simulink model "beta_inte"  (R2016b)
settings: Solver=FixedStepAuto  StartTime=0.0  StopTime=90  FixedStep=0.01  RelTol=1e-3
values from neighbouring files (symbols this model uses):
  T = 0.47    [Init_for_washout_filter.m]
settings Model: Creator=pallavr  LastModifiedBy=pallavr

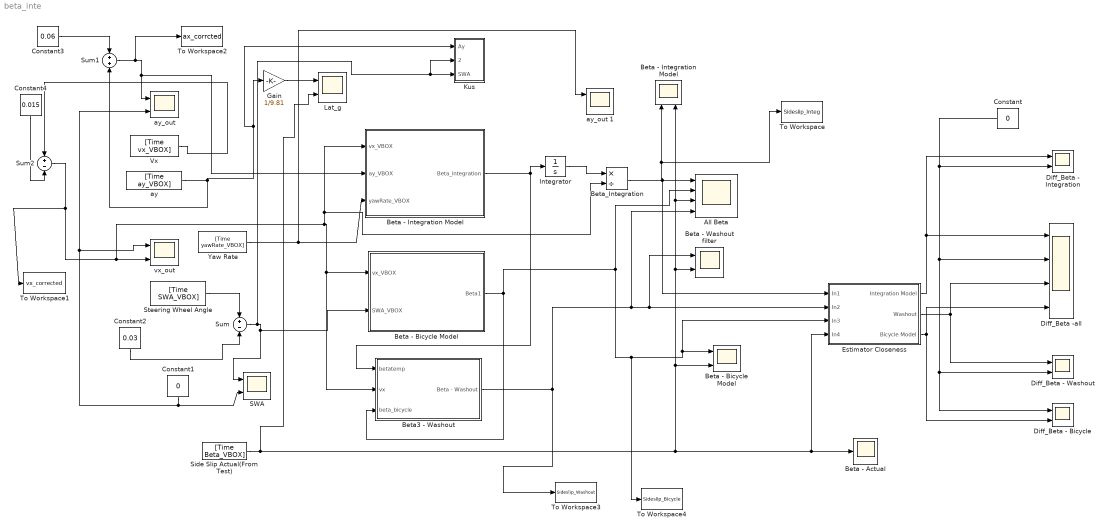
== system beta_inte ==
  " Beta - Bicycle Model" : Scope  NumInputPorts=2
  " Beta - Integration Model" : Scope  NumInputPorts=2
  " Beta - Washout filter" : Scope  NumInputPorts=2
  All Beta : Scope  NumInputPorts=4
  Beta - Actual : Scope
  Beta - Bicycle Model : MATLAB Function  TreatAsAtomicUnit=on
  Beta - Integration Model : MATLAB Function  TreatAsAtomicUnit=on
  "Beta3 - Washout " : Subsystem
  Beta_Integration : Product  Inputs=*/
  Constant : Constant  Value=0
  Constant1 : Constant  Value=0
  Constant2 : Constant  Value=0.03
  Constant3 : Constant  Value=0.06
  Constant4 : Constant  Value=0.015
  "Diff_Beta - Bicycle " : Scope  NumInputPorts=2
  Diff_Beta - Integration : Scope  NumInputPorts=2
  Diff_Beta - Washout : Scope  NumInputPorts=2
  Diff_Beta -all : Scope  NumInputPorts=4
  Estimator Closeness : Subsystem
  Gain : Gain  Gain=1/9.81
  Integrator : Integrator
  Kus : Subsystem
  Lat_g : Scope  NumInputPorts=2
  "SWA " : Scope  NumInputPorts=2
  Side Slip Actual(From Test) : FromWorkspace  VariableName=[Time Beta_VBOX]  SampleTime=0
  Steering Wheel Angle : FromWorkspace  VariableName=[Time SWA_VBOX]  SampleTime=0
  Sum : Sum  Inputs=+-
  Sum1 : Sum
  Sum2 : Sum  Inputs=+-
  To Workspace : ToWorkspace  VariableName=Sideslip_Integ  SampleTime=-1
  To Workspace1 : ToWorkspace  VariableName=vx_corrected  SampleTime=-1
  To Workspace2 : ToWorkspace  VariableName=ax_corrcted  SampleTime=-1
  To Workspace3 : ToWorkspace  VariableName=Sideslip_Washout  SampleTime=-1
  To Workspace4 : ToWorkspace  VariableName=Sideslip_Bicycle  SampleTime=-1
  Vx : FromWorkspace  VariableName=[Time vx_VBOX]  SampleTime=0
  Yaw Rate : FromWorkspace  VariableName=[Time yawRate_VBOX]  SampleTime=0
  ay : FromWorkspace  VariableName=[Time ay_VBOX]  SampleTime=0
  "ay_out " : Scope  NumInputPorts=2
  ay_out 1 : Scope  NumInputPorts=2
  "vx_out " : Scope  NumInputPorts=2
  wires:
  Integrator/1 -> Beta_Integration/1
  Beta - Bicycle Model/1(Beta1) -> Estimator Closeness/3(In3), " Beta - Bicycle Model"/1, To Workspace4/1, All Beta/2, "Beta3 - Washout "/3(beta_bicycle)
  Beta_Integration/1 -> Estimator Closeness/1(In1), All Beta/1, To Workspace/1, " Beta - Integration Model"/1
  Side Slip Actual(From Test)/1 -> Lat_g/2, " Beta - Integration Model"/2, All Beta/3, " Beta - Washout filter"/2, " Beta - Bicycle Model"/2, Beta - Actual/1, Estimator Closeness/4(In4)
  ay/1 -> Kus/1(Ay), Gain/1, Sum1/2
  Yaw Rate/1 -> Beta - Integration Model/3(yawRate_VBOX), ay_out 1/1
  Beta - Integration Model/1(Beta_integration) -> Integrator/1, "Beta3 - Washout "/1(betatemp)
  "Beta3 - Washout "/1(Beta - Washout) -> " Beta - Washout filter"/1, Estimator Closeness/2(In2), All Beta/4, To Workspace3/1
  Estimator Closeness/1(Integration Model) -> Diff_Beta - Integration/1, Diff_Beta -all/1
  Estimator Closeness/2("Washout ") -> Diff_Beta - Washout/1, Diff_Beta -all/3
  Constant/1 -> Diff_Beta - Integration/2, Diff_Beta -all/2, Diff_Beta - Washout/2, "Diff_Beta - Bicycle "/1
  Estimator Closeness/3(Bicycle Model) -> Diff_Beta -all/4, "Diff_Beta - Bicycle "/2
  Gain/1 -> Lat_g/1
  Steering Wheel Angle/1 -> Sum/1
  Constant1/1 -> "SWA "/2, "vx_out "/1, "ay_out "/2
  Vx/1 -> Sum2/1
  Constant2/1 -> Sum/2
  Constant3/1 -> Sum1/1
  Sum1/1 -> To Workspace2/1, Beta - Integration Model/2(ay_VBOX), "ay_out "/1
  Constant4/1 -> Sum2/2
  Sum2/1 -> To Workspace1/1, Beta_Integration/2, Beta - Integration Model/1(vx_VBOX), Beta - Bicycle Model/1(vx_VBOX), "Beta3 - Washout "/2(vx), "vx_out "/2
  Sum/1 -> Kus/2("SWA_in "), Kus/3(SWA), Beta - Bicycle Model/2(SWA_VBOX), "SWA "/1

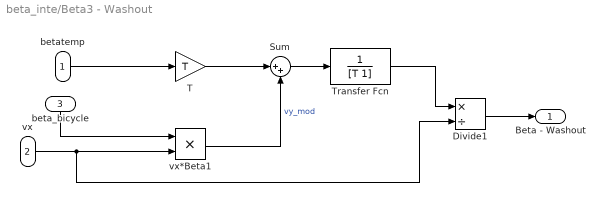
== system beta_inte/Beta3 - Washout  ==
  betatemp : Inport
  vx : Inport  Port=2
  beta_bicycle : Inport  Port=3
  Divide1 : Product  Inputs=*/
  Sum : Sum  Inputs=|++
  T : Gain  Gain=T
  Transfer Fcn : TransferFcn  Denominator=[T 1]
  vx*Beta1 : Product
  Beta - Washout : Outport
  wires:
  Sum/1 -> Transfer Fcn/1
  T/1 -> Sum/1
  Transfer Fcn/1 -> Divide1/1
  Divide1/1 -> Beta - Washout/1
  vx*Beta1/1 -> Sum/2  "vy_mod"
  vx/1 -> Divide1/2, vx*Beta1/2
  beta_bicycle/1 -> vx*Beta1/1
  betatemp/1 -> T/1

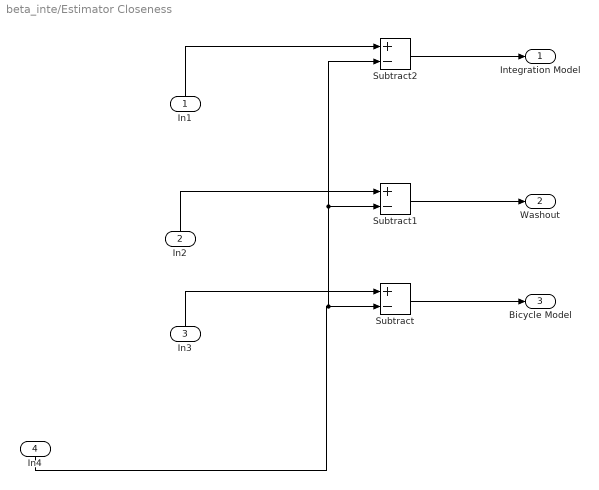
== system beta_inte/Estimator Closeness ==
  In1 : Inport
  In2 : Inport  Port=2
  In3 : Inport  Port=3
  In4 : Inport  Port=4
  Subtract : Sum  Inputs=+-
  Subtract1 : Sum  Inputs=+-
  Subtract2 : Sum  Inputs=+-
  Integration Model : Outport
  "Washout " : Outport  Port=2
  Bicycle Model : Outport  Port=3
  wires:
  Subtract2/1 -> Integration Model/1
  Subtract/1 -> Bicycle Model/1
  In3/1 -> Subtract/1
  In4/1 -> Subtract2/2, Subtract1/2, Subtract/2
  In2/1 -> Subtract1/1
  In1/1 -> Subtract2/1
  Subtract1/1 -> "Washout "/1

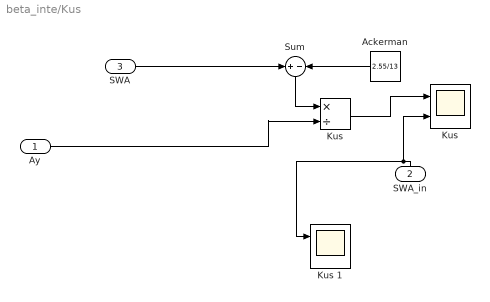
== system beta_inte/Kus ==
  Ay : Inport
  "SWA_in " : Inport  Port=2
  SWA : Inport  Port=3
  Ackerman : Constant  Value=2.55/13
  Kus : Product  Inputs=*/
  "Kus " : Scope  NumInputPorts=2
  Kus 1 : Scope  NumInputPorts=2
  Sum : Sum  Inputs=+-
  wires:
  Ackerman/1 -> Sum/2
  Kus/1 -> "Kus "/1
  Sum/1 -> Kus/1
  SWA/1 -> Sum/1
  Ay/1 -> Kus/2
  "SWA_in "/1 -> "Kus "/2, Kus 1/1

== matlab function beta_inte/Beta - Integration Model ==
  data: vx_VBOX input; Beta_integration output; ay_VBOX input; yawRate_VBOX input
function Beta_integration = fcn(vx_VBOX,ay_VBOX,yawRate_VBOX)

Beta_integration = (ay_VBOX.*(1-0.087))-(yawRate_VBOX.*vx_VBOX)

== matlab function beta_inte/Beta - Bicycle Model ==
  data: vx_VBOX input; Beta1 output; SWA_VBOX input
function Beta1 = fcn(vx_VBOX,SWA_VBOX)
lf=0.41*2.55;       % Distance from CoG to front axis (m)
lr=2.55-lf;         % Distance from CoG to rear axis (m)
L=lf+lr;            % Wheel base (m)
mass=1435-80;       % Mass (kg)
Ratio=17;           % Steering gear ratio
Cf=70000;          % Lateral stiffness front axle (N/rad) [FREE TO TUNE]
Cr=70000;          % Lateral stiffness rear axle (N/rad) [FREE TO TUNE]

Beta1 = ((lr.*L.*Cf.*Cr-lf.*Cf.*mass.*(vx_VBOX.^2)).*SWA_VBOX)./((Ratio).*(L*L*Cf*Cr+mass.*(vx_VBOX.^2).*(lr*Cr-lf*Cf)));
